simulink model "ControllerPID"  (R2021a)
settings: Solver=VariableStepAuto  StartTime=0.0  StopTime=0.1  RelTol=1e-3
values from neighbouring files (symbols this model uses):
  Bm = NoLoadTorque/NoLoadSpeed    [Script.m]
  CF = 1000    [Script.m]
  ExpectedSpeed = RPMtoRad(8000/83)    [Script.m]
  KLoad = 0.95    [Script.m]
  MinLoadTorque = 5*NoLoadTorque    [Script.m]
  sampleTime = 1e-6    (= 1e-06)    [Script.m]
undefined symbols (not defined in the file or in its folder): eff, GearBoxRatio, Jg, Jm, Kd, Ki, Km, Kp, Lw, Rw
libraries: pid_lib x1
settings Model: Creator=circl  LastModifiedBy=circl

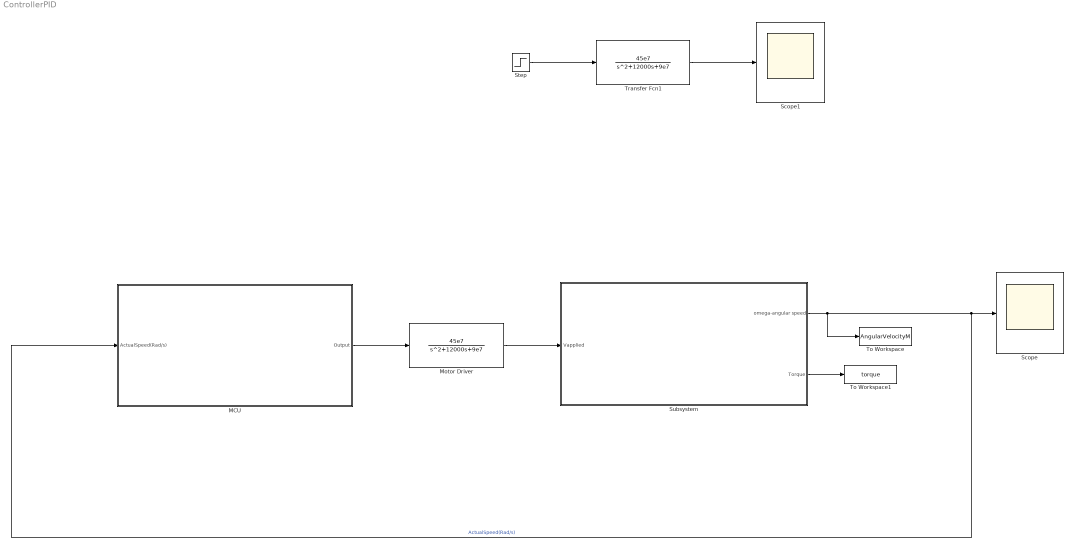
== system ControllerPID ==
  MCU : Subsystem
  Motor Driver : TransferFcn  Numerator=[45e7 ]  Denominator=[1 12000 9e7]
  Scope : Scope
  Scope1 : Scope
  Step : Step  Time=0  SampleTime=0
  Subsystem : Subsystem
  To Workspace : ToWorkspace  VariableName=AngularVelocityM  SaveFormat=Timeseries  SampleTime=sampleTime
  To Workspace1 : ToWorkspace  VariableName=torque  SaveFormat=Timeseries  SampleTime=-1
  Transfer Fcn1 : TransferFcn  Numerator=[45e7 ]  Denominator=[1 12000 9e7]
  wires:
  Subsystem/1(omega-angular speed) -> MCU/1(ActualSpeed(Rad/s)), Scope/1, To Workspace/1  "ActualSpeed(Rad/s)"
  Subsystem/2(Torque) -> To Workspace1/1
  Step/1 -> Transfer Fcn1/1
  Transfer Fcn1/1 -> Scope1/1
  MCU/1(Output) -> Motor Driver/1
  Motor Driver/1 -> Subsystem/1(Vapplied)

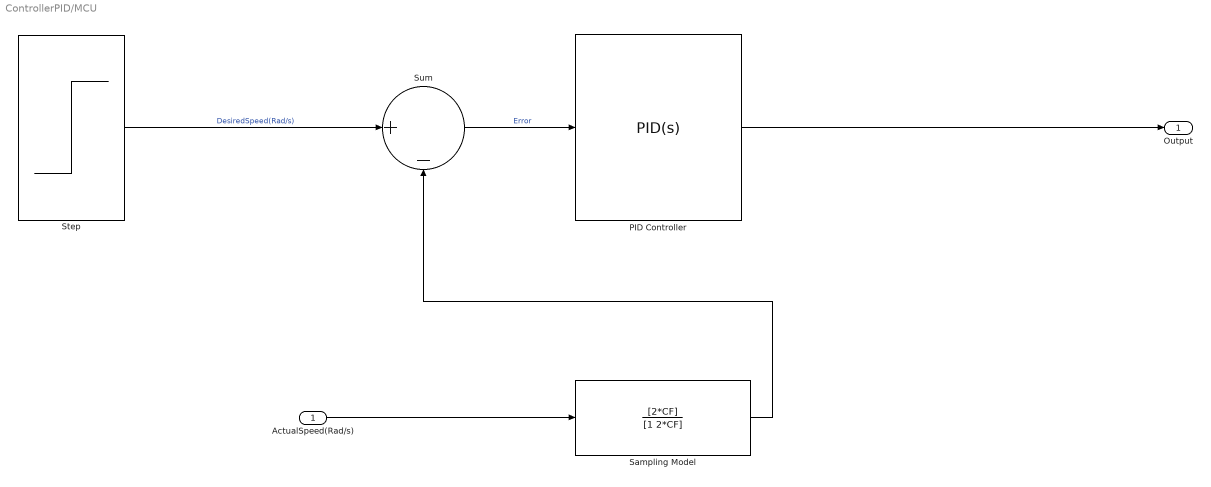
== system ControllerPID/MCU ==
  ActualSpeed(Rad/s) : Inport
  PID Controller : pid_lib/PID Controller  Controller=PID  Form=Parallel  TimeDomain=Continuous-time  UseExternalTs=off  SampleTime=-1  IntegratorMethod=Forward Euler  FilterMethod=Forward Euler  ControllerParametersSource=internal  P=Kp  I=Ki  D=Kd  UseFilter=on  N=100  TunerSelectOption=Transfer Function Based (PID Tuner App)  InitialConditionSource=internal  InitialConditionForIntegrator=0  InitialConditionForFilter=0  DifferentiatorICPrevScaledInput=0  ExternalReset=none  TrackingMode=off  Kt=1  LimitOutput=off  SatLimitsSource=internal  UpperSaturationLimit=inf  LowerSaturationLimit=-inf  LinearizeAsGain=on  AntiWindupMode=none  Kb=1  POutMin=[]  POutMax=[]  IOutMin=[]  IOutMax=[]  DOutMin=[]  DOutMax=[]  NOutMin=[]  NOutMax=[]  SumOutMin=[]  SumOutMax=[]  SaturationOutMin=[]  SaturationOutMax=[]  PParamMin=[]  PParamMax=[]  IParamMin=[]  IParamMax=[]  DParamMin=[]  DParamMax=[]  NParamMin=[]  NParamMax=[]  KbParamMin=[]  KbParamMax=[]  KtParamMin=[]  KtParamMax=[]  KbOutMin=[]  KbOutMax=[]  KtOutMin=[]  KtOutMax=[]  IntegratorOutMin=[]  IntegratorOutMax=[]  FilterOutMin=[]  FilterOutMax=[]  SumI1OutMin=[]  SumI1OutMax=[]  SumI2OutMin=[]  SumI2OutMax=[]  SumI3OutMin=[]  SumI3OutMax=[]  SumI4OutMin=[]  SumI4OutMax=[]  SumDOutMin=[]  SumDOutMax=[]  DifferentiatorOutMin=[]  DifferentiatorOutMax=[]  FilterDiffOutCoefMin=[]  FilterDiffOutCoefMax=[]  ReciprocalOutMin=[]  ReciprocalOutMax=[]  SumDenOutMin=[]  SumDenOutMax=[]  SumNumOutMin=[]  SumNumOutMax=[]  DivideOutMin=[]  DivideOutMax=[]  UdiffTsProdOutMin=[]  UdiffTsProdOutMax=[]  NTsProdOutMin=[]  NTsProdOutMax=[]  UintegralTsProdOutMin=[]  UintegralTsProdOutMax=[]  UngainTsProdOutMin=[]  UngainTsProdOutMax=[]  IntegratorContinuousStateAttributes=''  IntegratorStateMustResolveToSignalObject=off  IntegratorRTWStateStorageClass=Auto  FilterContinuousStateAttributes=''  FilterStateMustResolveToSignalObject=off  FilterRTWStateStorageClass=Auto  ParallelPVariant=InternalParameters  IdealPVariant=Disabled  IVariant=InternalParameters  DVariant=InternalParameters  IntegratorVariant=Continuous  SatVariant=Disabled  AWVariant=Passthrough  PCopyVariant=Disabled  TRVariant=Disabled  FdbkBlocksVariant=Forward  IdealPFdbkVariant=Disabled  SatFdbkVariant=Disabled  DerivativeFilterVariant=ContFilter  NVariant=InternalParameters  NCopyVariant=Disabled  FilterICVariant=InternalICsFilter  IntegratorICVariant=InternalICs  ExternalResetVariant=Disabled  TRSumVariant=Passthrough  SumFdbkVariant=Disabled  SumVariant=Sum_PID  TsampFilterVariant=InternalTs  TsampNgainVariant=Passthrough  TsampIntegralVariant=Passthrough  ExternalSaturationOutDataTypeStr=Inherit: Same as second input
  Sampling Model : TransferFcn  Numerator=[2*CF]  Denominator=[1 2*CF]
  Step : Step  Time=0  After=ExpectedSpeed  SampleTime=sampleTime
  Sum : Sum  Inputs=|+-
  Output : Outport
  wires:
  Step/1 -> Sum/1  "DesiredSpeed(Rad/s)"
  ActualSpeed(Rad/s)/1 -> Sampling Model/1
  Sum/1 -> PID Controller/1  "Error"
  Sampling Model/1 -> Sum/2
  PID Controller/1 -> Output/1

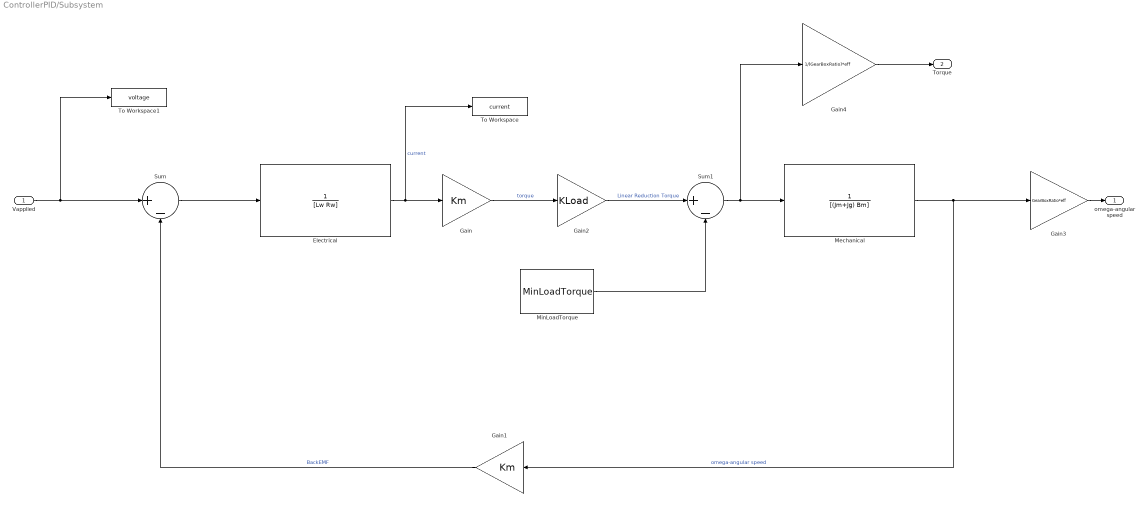
== system ControllerPID/Subsystem ==
  Vapplied : Inport
  Electrical : TransferFcn  Denominator=[Lw Rw]
  Gain : Gain  Gain=Km
  Gain1 : Gain  Gain=Km
  Gain2 : Gain  Gain=KLoad
  Gain3 : Gain  Gain=GearBoxRatio*eff
  Gain4 : Gain  Gain=1/(GearBoxRatio)*eff
  "Mechanical " : TransferFcn  Denominator=[(Jm+Jg) Bm]
  MinLoadTorque : Constant  Value=MinLoadTorque
  Sum : Sum  Inputs=|+-
  Sum1 : Sum  Inputs=|+-
  To Workspace : ToWorkspace  VariableName=current  SaveFormat=Timeseries  SampleTime=-1
  To Workspace1 : ToWorkspace  VariableName=voltage  SaveFormat=Timeseries  SampleTime=-1
  omega-angular speed : Outport
  Torque : Outport  Port=2
  wires:
  Electrical/1 -> To Workspace/1, Gain/1  "current"
  "Mechanical "/1 -> Gain1/1, Gain3/1  "omega-angular speed"
  Sum/1 -> Electrical/1
  Gain1/1 -> Sum/2  "BackEMF"
  Vapplied/1 -> To Workspace1/1, Sum/1
  Gain/1 -> Gain2/1  "torque"
  Sum1/1 -> Gain4/1, "Mechanical "/1
  Gain2/1 -> Sum1/1  "Linear Reduction Torque"
  MinLoadTorque/1 -> Sum1/2
  Gain3/1 -> omega-angular speed/1
  Gain4/1 -> Torque/1
